simulink model "Simulink"  (R2020b)
settings: Solver=VariableStepAuto  StartTime=0.0  StopTime=100  RelTol=1e-3
undefined symbols (not defined in the file): Am, Ap
settings Model: Creator=sokra  LastModifiedBy=sokra

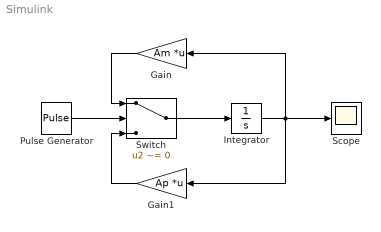
== system Simulink ==
  Gain : Gain  Gain=Am  Multiplication=Matrix(K*u)
  Gain1 : Gain  Gain=Ap  Multiplication=Matrix(K*u)
  Integrator : Integrator  InitialCondition=[1;1]
  Pulse Generator : DiscretePulseGenerator  PulseType=Time based  Period=0.1  PulseWidth=eps*100
  Scope : Scope
  Switch : Switch  Criteria=u2 ~= 0
  wires:
  Pulse Generator/1 -> Switch/2
  Switch/1 -> Integrator/1
  Gain/1 -> Switch/1
  Gain1/1 -> Switch/3
  Integrator/1 -> Gain1/1, Scope/1, Gain/1
